simulink model "lab4"  (R2020b)
settings: Solver=VariableStepAuto  StartTime=0.0  StopTime=4.1666666666261622E-8  RelTol=1e-10
libraries: simulink x1
settings Model: Creator=Le tueur  LastModifiedBy=Le tueur
settings SolverCC: MaxConsecutiveMinStep=100

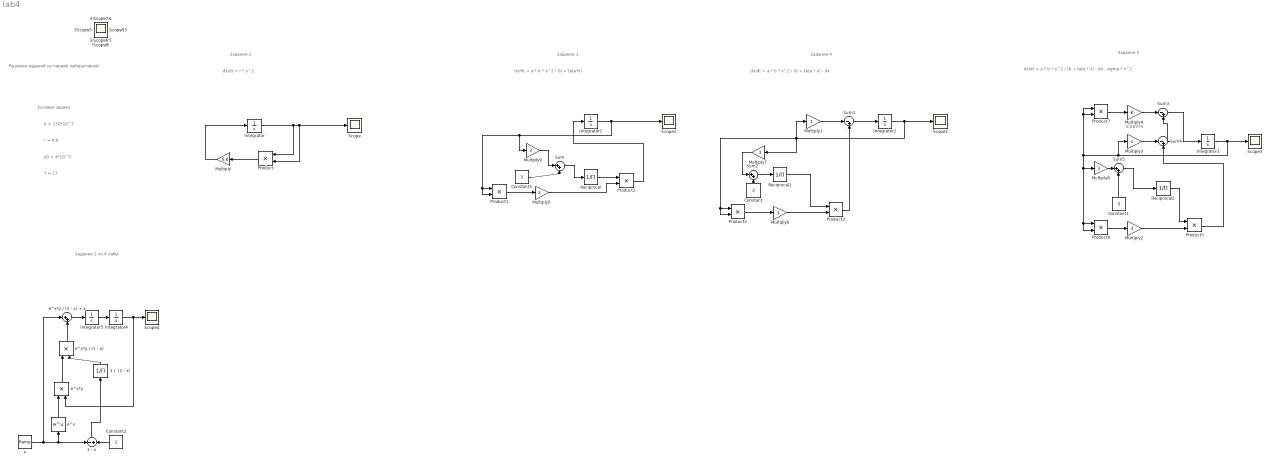
== system lab4 ==
  note: Задание 2 из 4 лабы
  note: Решения заданий из первой лабораторной
  note: dx/dt = a * b * x^2 / (b + teta * x) - dx - sigma * x^2
  note: dx/dt = a * b * x^2 / (b + teta * x) - dx
  note: Задание 5
  note: Задание 4
  note: dx/dt = a * b * x^2 / (b + teta*x)
  note: Задание 3
  note: dx/dt = r * x^2
  note: Задание 2
  note: T = 17
  note: y0 = 4*10^7
  note: r = 0.6
  note: K = 150*10^7
  note: Условие задачи
  1 - x : Sum  Inputs=-+
  1 /  (1 - x) : Product  Inputs=/
  Constant : Constant  Value=3
  Constant1 : Constant  Value=3
  Constant2 : Constant
  Constant3 : Constant  Value=3
  Integrator{,1..3} (4 alike) : Integrator  InitialCondition=4*10^7
  Integrator4 : Integrator
  Integrator5 : Integrator
  Multiply : Gain  Gain=0.6
  Multiply1 : Gain
  Multiply{2,5..9} (6 alike) : Gain  Gain=3
  Multiply3 : Gain
  Multiply4 : Gain  Gain=0.00575
  Product{,1..7} (8 alike) : Product
  Reciprocal : Product  Inputs=/
  Reciprocal1 : Product  Inputs=/
  Reciprocal2 : Product  Inputs=/
  Scope{,1..23} (24 alike) : Scope
  Sum : Sum  Inputs=|++
  Sum1 : Sum  Inputs=|-+
  Sum2 : Sum  Inputs=|++
  Sum3 : Sum  Inputs=|-+
  Sum4 : Sum  Inputs=|-+
  Sum5 : Sum  Inputs=|++
  e^x : Math  SaturateOnIntegerOverflow=on
  e^x*y : Product
  e^x*y / (1 - x) : Product
  e^x*y / (1 - x) + x : Sum  Inputs=|++
  x : simulink/Sources/Ramp  slope=1  start=0  InitialOutput=0
  wires:
  Integrator/1 -> Product/1, Product/2, Scope/1
  Multiply/1 -> Integrator/1
  Product/1 -> Multiply/1
  Integrator1/1 -> Multiply9/1, Product1/2, Product1/1, Scope1/1
  Integrator2/1 -> Multiply7/1, Product4/2, Product4/1, Multiply1/1, Scope2/1
  Multiply1/1 -> Sum1/1
  Sum1/1 -> Integrator2/1
  Constant/1 -> Sum2/2
  Sum2/1 -> Reciprocal1/1
  Reciprocal1/1 -> Product3/1
  Product3/1 -> Sum1/2
  Integrator3/1 -> Product7/1, Product7/2, Multiply8/1, Product6/1, Product6/2, Multiply3/1, Scope3/1
  Sum3/1 -> Integrator3/1
  Reciprocal2/1 -> Product5/1
  Product6/1 -> Multiply2/1
  Multiply2/1 -> Product5/2
  Sum4/1 -> Sum3/2
  Product5/1 -> Sum4/2
  Multiply3/1 -> Sum4/1
  Sum5/1 -> Reciprocal2/1
  Product7/1 -> Multiply4/1
  Multiply4/1 -> Sum3/1
  Integrator4/1 -> e^x*y/2, Scope4/1
  Integrator5/1 -> Integrator4/1
  x/1 -> e^x*y / (1 - x) + x/1, 1 - x/1, e^x/1
  Constant2/1 -> 1 - x/2
  e^x/1 -> e^x*y/1
  1 - x/1 -> 1 /  (1 - x)/1
  1 /  (1 - x)/1 -> e^x*y / (1 - x)/2
  e^x*y/1 -> e^x*y / (1 - x)/1
  e^x*y / (1 - x)/1 -> e^x*y / (1 - x) + x/2
  e^x*y / (1 - x) + x/1 -> Integrator5/1
  Product1/1 -> Multiply5/1
  Multiply5/1 -> Product2/2
  Reciprocal/1 -> Product2/1
  Product2/1 -> Integrator1/1
  Constant3/1 -> Sum/2
  Sum/1 -> Reciprocal/1
  Multiply9/1 -> Sum/1
  Product4/1 -> Multiply6/1
  Multiply6/1 -> Product3/2
  Multiply7/1 -> Sum2/1
  Constant1/1 -> Sum5/2
  Multiply8/1 -> Sum5/1
